simulink model "noise"  (R2019a)
settings: Solver=VariableStepAuto  StartTime=0.0  StopTime=2000.0  RelTol=1e-3
values from neighbouring files (symbols this model uses):
  A = [0 -4.5 0; 0 -0.025 0.000013;0 0 -5.54/60 ]    [Project.m]
  B = [0 0 1/12]'    [Project.m]
  C = [1 0 0]    [Project.m]
  D_bilinear = [D_bilinear;d{1}]    [Project.m]
  D_matched = [D_matched;d{1}]    [Project.m]
  N_bilinear = [N_bilinear;n{1}]    [Project.m]
  N_matched = [N_matched;n{1}]    [Project.m]
  Ts = [ 0.1 0.9 100]    [Project.m]
libraries: simulink x1
settings Model: Creator=atefeh  LastModifiedBy=atefeh

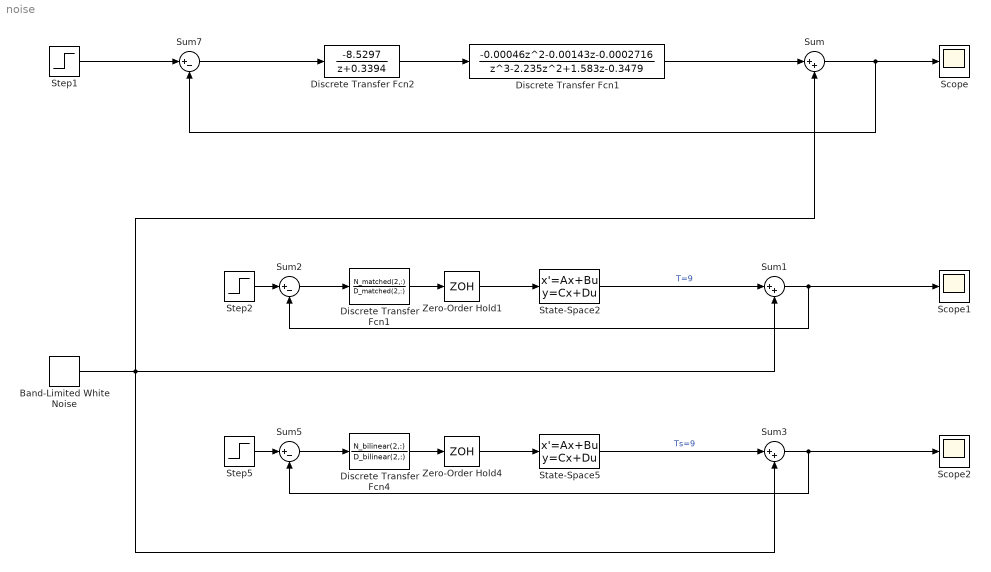
== system noise ==
  Band-Limited White Noise : simulink/Sources/Band-Limited White Noise  Cov=[0.001]  Ts=0.1  seed=[23341]
  Discrete Transfer Fcn1 : DiscreteTransferFcn  Numerator=N_matched(2,:)  Denominator=D_matched(2,:)  SampleTime=Ts(2)
  "Discrete Transfer Fcn1 " : DiscreteTransferFcn  Numerator=[-0.00046 -0.00143 -0.0002716]  Denominator=[1 -2.235 1.583 -0.3479]  SampleTime=9
  "Discrete Transfer Fcn2 " : DiscreteTransferFcn  Numerator=[-8.5297]  Denominator=[1 0.3394]  SampleTime=9
  Discrete Transfer Fcn4 : DiscreteTransferFcn  Numerator=N_bilinear(2,:)  Denominator=D_bilinear(2,:)  SampleTime=Ts(2)
  Scope : Scope
  Scope1 : Scope
  Scope2 : Scope
  State-Space2 : StateSpace  A=A  B=B  C=C  D=0  InitialCondition=0
  State-Space5 : StateSpace  A=A  B=B  C=C  D=0  InitialCondition=0
  "Step1 " : Step  SampleTime=0
  Step2 : Step  SampleTime=0
  Step5 : Step  SampleTime=0
  Sum : Sum  Inputs=|++
  Sum1 : Sum  Inputs=|++
  Sum2 : Sum  Inputs=|+-
  Sum3 : Sum  Inputs=|++
  Sum5 : Sum  Inputs=|+-
  Sum7 : Sum  Inputs=|+-
  Zero-Order Hold1 : ZeroOrderHold  SampleTime=-1
  Zero-Order Hold4 : ZeroOrderHold  SampleTime=-1
  wires:
  "Step1 "/1 -> Sum7/1
  "Discrete Transfer Fcn1 "/1 -> Sum/1
  Sum7/1 -> "Discrete Transfer Fcn2 "/1
  "Discrete Transfer Fcn2 "/1 -> "Discrete Transfer Fcn1 "/1
  Sum/1 -> Sum7/2, Scope/1
  Zero-Order Hold1/1 -> State-Space2/1
  Discrete Transfer Fcn1/1 -> Zero-Order Hold1/1
  Step2/1 -> Sum2/1
  State-Space2/1 -> Sum1/1  "T=9"
  Sum2/1 -> Discrete Transfer Fcn1/1
  State-Space5/1 -> Sum3/1  "Ts=9"
  Zero-Order Hold4/1 -> State-Space5/1
  Discrete Transfer Fcn4/1 -> Zero-Order Hold4/1
  Sum5/1 -> Discrete Transfer Fcn4/1
  Step5/1 -> Sum5/1
  Sum1/1 -> Scope1/1, Sum2/2
  Band-Limited White Noise/1 -> Sum1/2, Sum3/2, Sum/2
  Sum3/1 -> Scope2/1, Sum5/2
